simulink model "model_part1"  (R2019b)
settings: Solver=FixedStepAuto  StartTime=0.0  StopTime=20  FixedStep=0.01  RelTol=1e-3
libraries: simulink x1
settings Model: Creator=Pc  LastModifiedBy=Pc
settings DataIOCC: ReturnWorkspaceOutputs=off

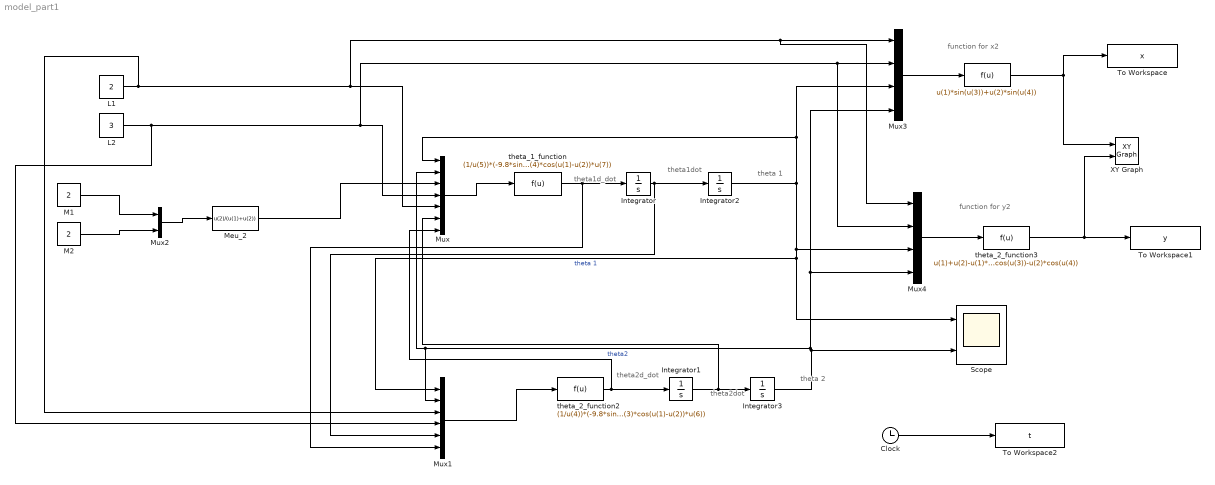
== system model_part1 ==
  note: function for y2
  note: function for x2
  note: theta1d_dot
  note: theta 1
  note: theta1dot
  note: theta 2
  note: theta2dot
  note: theta2d_dot
  " " : Fcn  Expr=u(1)*sin(u(3))+u(2)*sin(u(4))
  Clock : Clock
  Integrator : Integrator  ContinuousStateAttributes='xdot'
  Integrator1 : Integrator  ContinuousStateAttributes='xdot'
  Integrator2 : Integrator  InitialCondition=pi/2  ContinuousStateAttributes='x'
  Integrator3 : Integrator  InitialCondition=pi/2  ContinuousStateAttributes='x'
  L1 : Constant  Value=2
  L2 : Constant  Value=3
  M1 : Constant  Value=2
  M2 : Constant  Value=2
  Meu_2 : Fcn  Expr=u(2)/(u(1)+u(2))
  Mux : Mux  Inputs=7
  Mux1 : Mux  Inputs=6
  Mux2 : Mux  Inputs=2
  Mux3 : Mux
  Mux4 : Mux
  Scope : Scope  NumInputPorts=2
  To Workspace : ToWorkspace  VariableName=x  SampleTime=-1
  To Workspace1 : ToWorkspace  VariableName=y  SampleTime=-1
  To Workspace2 : ToWorkspace  VariableName=t  SampleTime=-1
  XY Graph : simulink/Sinks/XY Graph  xmin=-6  xmax=6  ymin=0  ymax=6  st=-1
  theta_1_function : Fcn  Expr=(1/u(5))*(-9.8*sin(u(1))- u(3)*u(4)*sin(u(1)-u(2))*u(6)^2-u(3)*u(4)*cos(u(1)-u(2))*u(7))
  theta_2_function2 : Fcn  Expr=(1/u(4))*(-9.8*sin(u(2))+u(3)*sin(u(1)-u(2))*u(5)^2-u(3)*cos(u(1)-u(2))*u(6))
  theta_2_function3 : Fcn  Expr=u(1)+u(2)-u(1)*cos(u(3))-u(2)*cos(u(4))
  wires:
  Mux/1 -> theta_1_function/1
  Integrator2/1 -> Mux4/3, Mux1/1, Scope/1, Mux3/3, Mux/1  "theta 1"
  Integrator1/1 -> Mux/6, Integrator3/1
  theta_2_function2/1 -> Integrator1/1, Mux/7
  Mux1/1 -> theta_2_function2/1
  Mux2/1 -> Meu_2/1
  M1/1 -> Mux2/1
  M2/1 -> Mux2/2
  Meu_2/1 -> Mux/3
  L1/1 -> Mux1/3, Mux4/1, Mux3/1, Mux/5
  L2/1 -> Mux1/4, Mux4/2, Mux3/2, Mux/4
  Integrator/1 -> Mux1/5, Integrator2/1
  theta_1_function/1 -> Mux1/6, Integrator/1
  Mux3/1 -> " "/1
  Mux4/1 -> theta_2_function3/1
  " "/1 -> XY Graph/1, To Workspace/1
  theta_2_function3/1 -> XY Graph/2, To Workspace1/1
  Integrator3/1 -> Mux4/4, Mux3/4, Mux1/2, Mux/2, Scope/2  "theta2"
  Clock/1 -> To Workspace2/1
